simulink model "code_gen_man_bin"  (Simulink 7.5)
settings: Solver=FixedStepDiscrete  SolverMode=SingleTasking  StartTime=0.0  StopTime=10.0  FixedStep=0.01  RelTol=1e-3
InitFcn:
  | boat_constants
values from neighbouring files (symbols this model uses):
  figure8_waypoints = int32([ ... (first row only)    [boat_constants.m]
  InitialPoint = 0    [boat_constants.m]    (also in l2plus.m)
  IPStar = 0    [boat_constants.m]    (also in l2plus.m)
  ISA_g = 9.815    [boat_constants.m]
  MaxDwnPthStar = 1    [boat_constants.m]    (also in l2plus.m)
  OC2max = 49999    [boat_constants.m]    (also in simulation_constants.m)
  sampling_waypoints = int32([ ... (first row only)    [boat_constants.m]
  switchDistance = 4    [boat_constants.m]    (also in l2plus.m)
  T_step = 0.01    [boat_constants.m]    (also in common.m)
  tanIntercept = tan( 45*pi/180 )    [boat_constants.m]    (also in l2plus.m)
  test_waypoints = int32([ ... (first row only)    [boat_constants.m]
  TStar = single(4.5)    [boat_constants.m]    (also in l2plus.m = single(2))
  Turn2Track = 0    [boat_constants.m]    (also in l2plus.m)
  wheelbase = 3.27    [boat_constants.m]
undefined symbols (not defined in the file or in its folder): clearGpsData, clearSensorData, cpInitCommunications, DataEEInitAndClear, DataEEWrite, DiscIntNeverNeededParam, ecan1_buffered_transmit_matlab, ecan1_error_status_matlab, ecan1_init, GetAirData, getGpsData, getRevoData, getSensorData, GetThrottleData, GetWaterData, GetWindData, Init_onlyOnce, Init_Reset, initCalibrationRange, initGps, processNewCommData, processNewGpsData, processNewRevoData, setHilMode, u1, u2, uart1EnqueueStateData, uart2EnqueueActuatorData, y1
libraries: simulink x80, dsPICdrivers x50, uSimLib x4, simulink_need_slupdate x4
(part 6 of 6)

== matlab function Controller/Autonomous Controller/Rudder Command/L2 Plus ref WP1 ==
  data: reset input double; L2Vec output single; waypoints input int16; mode input uint8; Puav input single size=3; Vxyz input single size=3; switchDistance parameter double size=1; ISA_g parameter double; tanIntercept parameter double; MaxDwnPthStar parameter double; Turn2Track parameter double; InitialPoint parameter double; IPStar parameter double; TStar parameter double; as_c output single; i0 output double; i1 output double; WP0 output double; WP1 output double
function [L2Vec, as_c, i0, i1, WP0, WP1] = L2PlusWP1(reset, waypoints, mode, Puav, Vxyz, switchDistance, ...
    ISA_g, tanIntercept, MaxDwnPthStar,Turn2Track,...
    InitialPoint, IPStar, TStar)
%==============================
%     computes bank angle command for following a straight line
%     by creating an aim point that may be more than L2 away 
%     from the UAV. The aim point is (usually) farther along the path 
%     toward WP1 than the UAV, and the intercept
%     angle is less than or equal to a specified value. This limits the intercept
%     angle even when the UAV is within L2 of the path.
%     See L2PlusWP1.m for details
    
%         INPUTS   
%             T1      unit vector WP0-->WP1
%             N1      normal to T1
%             WP0     position of "from" waypoint. only needed to set an InitialPoint
%             WP1     position of WP1, active waypoint
%             Puav    position of UAV
%             Vxyz    Inertial velocity
%             switchDistance distance from WP1 to switch to WP2

%         PARAMETERS
%             ISA_g   gravity
%             tanIntercept  tangent of intercept angle
%             MaxDwnPthStar L2 multiplier to determmine downpath aimpoint
%             Turn2Track    true to turn toward T1 instead of L2
%             InitialPoint  true if no line tracking at first--fly direct to some initial point
%             IPStar        L2 multiplier to determing distance of IP from first WP0
%             Tstar         was called L2Base, time constant of response
%             
%         OUTPUTS
%             phi_c   commanded bank angle (positive is a starboard turn)
%             L2Vec   L2 vector toward aim point
%             as_c    commanded lateral acceleration
%             Groundspeed 
%             IP1     position of IP for plotting purposes. IP1(3) = -999 if no IP exists

    persistent IPActive;  %true if flying toward IP
    persistent IP; % location of initial point

    persistent index_0 index_1; % Store the indices for waypoints 0 & 1 respectively
    persistent direction; % Keep track of the direction for patrol mode
    
    % Make sure we have at least two waypoints
    assert(size(waypoints,1) >= 2);

    % Inititalize to the first waypoint
    if isempty(index_0)
        index_0 = int8(1);
    end
    if isempty(index_1)
        index_1 = int8(2);
    end
    if isempty(direction)
        direction = int8(1);
    end
    
    % Reset the waypoints
    if (reset)
        index_0 = int8(1);
        index_1 = int8(2);
    end
    
    % Select the two current waypoints we're dealing with
    WP0 = single(waypoints(index_0,:)');
    WP1 = single(waypoints(index_1,:)');
    i0 = index_0;
    i1 = index_1;
    
    switchToNextWaypoint = false;
    Pwp1 = single(zeros(3,1));
    Pe_y = single(0);
    Dist2WP1 = single(0);
    MinDownPath = single(0);
    Dist2WPSwitch = single(0);
    L2DownPath = single(0);
    L2ToT = single(zeros(3,1));
    L2Vec = single(zeros(3,1));
    IP1 = single([0; 0;-999]); %signal for no IP
    
    Pne = [Puav(1); Puav(2); 0]; %horizontal position
    Vne = [Vxyz(1); Vxyz(2); 0]; % horizontal velocity
    Groundspeed = norm(Vne);
    L2 = single(TStar*Groundspeed);
    WP0ne = single(zeros(3,1));
    
% Calculate N1 and T1
assert(norm(WP1 - WP0) ~= 0);
T1 = WP1-WP0;
T1 = T1/norm(T1);
N1 = [-T1(2); T1(1); 0];
    
%     initialize IP
    if (isempty(IPActive))
        if (InitialPoint)
%             IP is set relative to the first "from" waypoint
            IPActive = -1;
            IP = [WP0(1); WP0(2); 0] - L2*IPStar*T1;
            
            if (norm(IP-Pne) < .001)
                IPActive = 0;
                IP = single([0; 0; -999]);
            end
        else
            IPActive = 0;
            IP = single([0; 0;-999]); %signal for no IP
        end
    end
    IP1 = IP;
    
    
    if (IPActive)
%         no line tracking, direct to IP
        L2Vec = L2*(IP - Pne)/norm(IP - Pne);
%         check to see if at the IP to terminate this mode
        if norm(IP - Pne) < .1*L2
            IPActive = 0;
        end
    else
         if (Pne(1) < 2)
             IP1 = IP1;
         end
%         IP not active, track WP lines
        WPOne = [WP1(1); WP1(2); 0];
        Pwp1 = Pne - [WP1(1); WP1(2); 0]; % position of UAV relative to WP1
        Pe_y = single(Pwp1'*N1); % cross track error
        Dist2WP1 = -single(Pwp1'*T1); % distance to WP1

%         minimum down path distance for Aim Point intersection on T
%         is determined by the intercept angle but limited 
%         in case of very distant intecepts to MaxDwnPthStar*L2
        MinDownPath = single ( min( abs(Pe_y)/tanIntercept, MaxDwnPthStar*L2)); 
        Dist2WPSwitch = Dist2WP1 - switchDistance;
        if ( abs(Pe_y) > L2 )
    %             Make sure aimpoint is no closer to waypoint than calculated switch point.
            L2DownPath = MinDownPath;
        else
    %             within L2 of T and Dist2WPSwitch >= 0, but limit angle of L2 wrt T
            L2DownPath = (max(MinDownPath, (sqrt( L2^2 - Pe_y^2 ))));
        end
        
        if ( Dist2WPSwitch < 0 )
            switchToNextWaypoint = true;
        end
        
         % vector from Pwp1 to aim point on T1
         L2ToT = single(( Dist2WP1 - L2DownPath )*(-T1) - Pwp1);
         if (norm(L2ToT) < .001)
             L2Vec = L2*T1;
         else
            L2Vec = single(L2*( L2ToT/norm(L2ToT) )); % limit size to L2
         end
    %         L2Vec = L2ToT;
%         dummy statements
    end
    Zprod = single(Vxyz(1)*L2Vec(2) - Vxyz(2)*L2Vec(1)); %Z component of cross product
    sinEta = single(Zprod/(Groundspeed*L2));

    as_c = single(2*Groundspeed^2/(L2)*sinEta);
%         bank angle limits outside of this block
    phi_c = single(atan(as_c/ISA_g));

%         now override bank angle if heading in the wrong direction
    if ( Turn2Track && Dist2WPSwitch > 0 && ~IPActive ) 
%             turn to track not L2, gives min displacement from track
        if ( T1'*Vxyz < 0 )
            if ( Pe_y > 0 )
                phi_c = single(+pi/2);
                as_c = single(99);
            else
                phi_c = single(-pi/2);
                as_c = single(-99);
            end
        end
     else
%           turn toward L2, give min displacement toward WP0
        if ( L2Vec'*Vxyz < 0 )
            if ( sinEta < 0 )
                phi_c = single(-pi/2); 
                as_c = single(-99);
            else
                phi_c = single(+pi/2);
                as_c = single(99);
            end
        end
    end

% Now we process waypoint switching. This relies on the switchTrigger
% value set in the above L2+ controller code.
theEnd = false;
if index_1 + 1 <= size(waypoints,1) && waypoints(index_1+1,1) == -1 ...
                                    && waypoints(index_1+1,2) == -1 ...
                                    && waypoints(index_1+1,3) == -1
    theEnd = true;
end
if switchToNextWaypoint
    switch mode
        case 0 % Halt mode
            if size(waypoints,1) >= index_1 + 1 && ~theEnd
                index_0 = index_1;
                index_1 = index_1 + 1;
            end
        case 1 % Loop mode
            % We either continue moving forward through the waypoints...
            if size(waypoints,1) >= index_1 + 1 && ~theEnd
                index_0 = index_1;
                index_1 = index_1 + 1;
            % Or we wrap-around to the starting waypoint
            else
                index_0 = index_1;
                index_1 = int8(1);
            end
        case 2 % Patrol mode
            if direction == 1 % For the forwards direction
                % We either continue moving forwards through the waypoints...
                if size(waypoints,1) >= index_1 + 1 && ~theEnd
                    index_0 = index_1;
                    index_1 = index_1 + 1;
                % Or we start to go backwards
                else
                    index_0 = index_1;
                    index_1 = index_1 - 1;
                    direction = int8(0);
                end
            elseif direction == 0 % For the reverse direction
                % We either continue moving backwards through the waypoints...
                if index_1 - 1 >= 1
                    index_0 = index_1;
                    index_1 = index_1 - 1;
                % Or we start to go forwards
                else
                    index_0 = index_1;
                    index_1 = index_1 + 1;
                    direction = int8(1);
                end
            end
    end
end

== matlab function Actuator Outputs/To Drive Motor/myMux ==
  data: u1 input double; y output double; u2 input double; u3 input double; u4 input double; u5 input double
function y = myMux(u1, u2, u3, u4, u5)
u5_u16 = uint16(u5);
y = uint16([u1(1); u2(1); u3(1); u4(1); 0; 0; 0; 0;]);

len = length(u5);
if len > 1
    y(5) = bitor(bitshift(u5_u16(1),8),u5_u16(2));
elseif len > 0
    y(5) = u5_u16(1);
end
if len > 3
    y(6) = bitor(bitshift(u5_u16(3),8),u5_u16(4));
elseif len > 2
    y(6) = u5_u16(3);
end
if len > 5
    y(7) = bitor(bitshift(u5_u16(5),8),u5_u16(6));
elseif len > 4
    y(7) = u5_u16(5);
end
if len > 7
    y(8) = bitor(bitshift(u5_u16(7),8),u5_u16(8));
elseif len > 6
    y(8) = u5_u16(7);
end

== matlab function Sensor Inputs/GPS/Unpack sensor data ==
  data: latitude output double; longitude output double; altitude output double; year output double; month output double; day output double; hour output double; minute output double; second output double; cog output double; sog output double; u input uint8; hdop output double; fix output double; satellites output double; newGpsData output double
function [latitude, longitude, altitude, year, month, day, hour, minute, second, cog, sog, hdop, fix, satellites, newGpsData] = unpack(u)
%#eml

latitude = typecast(u(1:4), 'single');
longitude = typecast(u(5:8), 'single');
altitude = typecast(u(9:12), 'single');
year = u(13);
month = u(14);
day = u(15);
hour = u(16);
minute = u(17);
second = u(18);
cog = typecast(u(19:22), 'single');
sog = typecast(u(23:26), 'single');
hdop = typecast(u(27:30), 'single');
fix = u(31);
satellites = u(32);
newGpsData = u(33);

== matlab function Sensor Inputs/Estop detection/Unpack throttle data ==
  data: u input uint8; throttle output double; newData output double
function [throttle, newData] = unpack(u)
%#eml

throttle = typecast(u(1:2), 'int16');
newData = u(3);

== matlab function Sensor Inputs/Toggle ==
  data: u input double; y output double
function y = toggle(u)
%#eml

persistent pre_output;

% Initialize pre_output
if isempty(pre_output)
    pre_output = false;
end

% If we receive the toggle input, toggle
if u
    if pre_output
        pre_output = false;
    else
        pre_output = true;
    end
end

y = pre_output;

== matlab function Controller/Radio Control Inputs1/Detect calibration trigger/Compute Calibration State ==
  data: trigger input boolean; state output uint8; restoredCalibration input double
function state = fcn(trigger, restoredCalibration)
%#eml

persistent countdownTimer transitionCounter internalState;

% Initialize persistent variables
if isempty(countdownTimer)
    countdownTimer = uint8(0);
    transitionCounter = uint8(0);
    
    if restoredCalibration
        internalState = uint8(3);
    else
        internalState = uint8(0);
    end
end

% Do the state processing:
switch internalState
    case 0 % Off
        % When we get a trigger, go into state 1 clearing the timer for use
        if trigger
            transitionCounter = uint8(1);
            internalState = uint8(1);
            countdownTimer = uint8(0);
        end
    case 1 % Transition mode
        % Here we just keep a timer going and once it expires we go back to off,
        % otherwise we count transitions until we've hit 3 then we go to calibration mode.
        countdownTimer = countdownTimer + 1;
        if countdownTimer > 150
            internalState = uint8(0);
        elseif trigger
            transitionCounter = transitionCounter + 1;
        
            % Once we've hit three transitions, we're in calibration mode!
            if transitionCounter == uint8(3)
                internalState = uint8(2);
            end
        end
    case 2 % Calibration mode
        % On the trigger, go into a calibrated mode.
        if trigger
            internalState = uint8(3);
        end
    case 3 % Calibrated
        % When we get a trigger, go into state 4 clearing the timer for use
        if trigger
            transitionCounter = uint8(1);
            internalState = uint8(4);
            countdownTimer = uint8(0);
        end
    case 4 % Transition mode (post-calibration)
        % Here we just keep a timer going and once it expires we go back to calibrated,
        % otherwise we count transitions until we've hit 3 then we go to calibration mode.
        countdownTimer = countdownTimer + 1;
        if countdownTimer > 150
            internalState = uint8(3);
        elseif trigger
            transitionCounter = transitionCounter + 1;
        
            % Once we've hit three transitions, we're in calibration mode!
            if transitionCounter == uint8(3)
                internalState = uint8(2);
            end
        end
end

% Output the internal state
state = internalState;

== matlab function Sensor Inputs/Unpack wind data ==
  data: speed output double; direction output double; newData output double; u input uint8
function [speed, direction, newData] = unpack(u)
%#eml

speed = typecast(u(1:4), 'single');
direction = typecast(u(5:8), 'single');
newData = u(9);

== matlab function Controller/Select current waypoint track ==
  data: reset output double; nextTrack input double; resetTrackNumber input double; test_waypoints parameter double; figure8_waypoints parameter double; sampling_waypoints parameter double; waypoints output double
function [reset, waypoints] = selectTrack(nextTrack, resetTrackNumber, test_waypoints, figure8_waypoints, sampling_waypoints)
%#eml


% Initialize trackNumber.
% This variable is our state, which is the set of waypoints we're navigating
% between.
persistent trackNumber;
if isempty(trackNumber)
    trackNumber = uint8(1);
end

% Here is the logic for switching tracks. trackReset resets the trackNumber
% and nextTrack increments the track number
if resetTrackNumber
    trackNumber = uint8(1);
    reset = true;
elseif nextTrack
    trackNumber = trackNumber + uint8(1);
    if trackNumber > 3
        trackNumber = uint8(1);
    end
    reset = true;
else
    reset = false;
end

% 1 is for the test waypoints, 2 is for the figure eight, and 3 is
% for the data gathering waypoints.
switch trackNumber
    case 1
        waypoints = test_waypoints;
    case 2
        waypoints = figure8_waypoints;
    case 3
        waypoints = sampling_waypoints;
    otherwise
        waypoints = zeros(size(test_waypoints), 'int32');
end

== matlab function Transmit state data via UART1/Pack1 ==
  data: L2 input double; gPos input double; head input double; lPos input double; vel input double; wp0 input double; wp1 input double; y output double; rudder_pot input double; port_limit input double; sb_limit input double; lat input double; lon input double; alt input double; yr input double; mon input double; day input double; hr input double; min input double; sec input double; cog input double; sog input double; hdop input double; fix input double; sat input double; reset input double; load input double; rudder_angle input double; v_rpm input double; status input double; ordering input double; rudderAngleCommand input double; throttleCommand input double; batteryVoltage input double; batteryAmperage input double; lowRudderCalLimit input double; highRudderCalLimit input double; revoHeading input double; revoMagStatus input double; revoPitch input double; revoPitchStatus input double; revoRoll input double; revoRollStatus input double; revoDip input double; revoMagneticMagnitude input double; windSpeed input double; windDirection input double; airTemp input double; airPressure input double; airHumidity input double; waterSpeed input double; waterTemp input double; waterDepth input double
function y = fcn(L2, gPos, head, lPos, vel, wp0, wp1, rudder_pot, port_limit, sb_limit, lat, lon, alt, yr, mon, day, hr, min, sec, cog, sog, hdop, fix, sat, reset, load, rudder_angle, v_rpm, status, ordering, rudderAngleCommand, throttleCommand, batteryVoltage, batteryAmperage, lowRudderCalLimit, highRudderCalLimit, revoHeading, revoMagStatus, revoPitch, revoPitchStatus, revoRoll, revoRollStatus, revoDip, revoMagneticMagnitude, windSpeed, windDirection, airTemp, airPressure, airHumidity, waterSpeed, waterTemp, waterDepth)
%#eml

y = zeros(153, 1, 'uint8');
y(1:4) = packUint32BE(typecast(L2(1),'uint32'));
y(5:8) = packUint32BE(typecast(L2(2),'uint32'));
y(9:12) = packUint32BE(typecast(gPos(1),'uint32'));
y(13:16) = packUint32BE(typecast(gPos(2),'uint32'));
y(17:20) = packUint32BE(typecast(head,'uint32'));
y(21:24) = packUint32BE(typecast(lPos(1),'uint32'));
y(25:28) = packUint32BE(typecast(lPos(2),'uint32'));
y(29:32) = packUint32BE(typecast(vel(1),'uint32'));
y(33:36) = packUint32BE(typecast(vel(2),'uint32'));
y(37:40) = packUint32BE(typecast(wp0(1),'uint32'));
y(41:44) = packUint32BE(typecast(wp0(2),'uint32'));
y(45:48) = packUint32BE(typecast(wp1(1),'uint32'));
y(49:52) = packUint32BE(typecast(wp1(2),'uint32'));
y(53:54) = packUint16BE(rudder_pot);
y(55) = port_limit;
y(56) = sb_limit;
y(57:60) = packUint32BE(typecast(lat,'uint32'));
y(61:64) = packUint32BE(typecast(lon,'uint32'));
y(65:68) = packUint32BE(typecast(alt,'uint32'));
y(69) = yr;
y(70) = mon;
y(71) = day;
y(72) = hr;
y(73) = min;
y(74) = sec;
y(75:78) = packUint32BE(typecast(cog,'uint32'));
y(79:82) = packUint32BE(typecast(sog,'uint32'));
y(83:86) = packUint32BE(typecast(hdop,'uint32'));
y(87) = fix;
y(88) = sat;
y(89) = reset;
y(90) = load;
y(91:94) = packUint32BE(typecast(rudder_angle,'uint32'));
y(95:96) = packUint16BE(typecast(v_rpm,'uint16'));
y(97) = status;
y(98) = ordering;
y(99:102) = packUint32BE(typecast(rudderAngleCommand,'uint32'));
y(103:104) = packUint16BE(typecast(throttleCommand, 'uint16'));
y(105:108) = packUint32BE(typecast(batteryVoltage,'uint32'));
y(109:112) = packUint32BE(typecast(batteryAmperage,'uint32'));
y(113:114) = packUint16BE(typecast(lowRudderCalLimit, 'uint16'));
y(115:116) = packUint16BE(typecast(highRudderCalLimit, 'uint16'));
y(117:120) = packUint32BE(typecast(revoHeading,'uint32'));
y(121) = revoMagStatus;
y(122:125) = packUint32BE(typecast(revoPitch,'uint32'));
y(126) = revoPitchStatus;
y(127:130) = packUint32BE(typecast(revoRoll,'uint32'));
y(131) = revoRollStatus;
y(132:135) = packUint32BE(typecast(revoDip, 'uint32'));
y(136:137) = packUint16BE(typecast(revoMagneticMagnitude,'uint16'));
y(138:139) = packUint16BE(typecast(windSpeed, 'uint16'));
y(140:141) = packUint16BE(typecast(windDirection, 'uint16'));
y(142:143) = packUint16BE(typecast(airTemp, 'uint16'));
y(144:145) = packUint16BE(typecast(airPressure, 'uint16'));
y(146:147) = packUint16BE(typecast(airHumidity, 'uint16'));
y(148:149) = packUint16BE(typecast(waterSpeed, 'uint16'));
y(150:151) = packUint16BE(typecast(waterTemp, 'uint16'));
y(152:153) = packUint16BE(typecast(waterDepth, 'uint16'));

function out = packUint32BE(in)
out = zeros(4, 1, 'uint8');
out(1) = uint8(bitand(bitshift(in,-24),hex2dec('FF')));
out(2) = uint8(bitand(bitshift(in,-16),hex2dec('FF')));
out(3) = uint8(bitand(bitshift(in,-8),hex2dec('FF')));
out(4) = uint8(bitand(in,hex2dec('FF')));

function out = packUint16BE(in)
out = zeros(2, 1, 'uint8');
out(1) = uint8(bitand(bitshift(in,-8),hex2dec('FF')));
out(2) = uint8(bitand(in,hex2dec('FF')));

== matlab function Controller/Radio Control Inputs1/If Action Subsystem1/Map into range ==
  data: mappedValue output int32; val input int32; in_min input int32; in_max input int32; out_min input int32; out_max input int32
function mappedValue = map(val, in_min, in_max, out_min, out_max)
%#eml
% Pulled from: http://www.arduino.cc/cgi-bin/yabb2/YaBB.pl?num=1289758376, first post
% This is a basic integer implementation of a map() function.
% NOTE: There can be integer overflow in the first multiplication.

  mappedValue = (val - in_min) * (out_max - out_min) / (in_max - in_min) + out_min;

end

== matlab function Controller/Radio Control Inputs1/If Action Subsystem3/Map into range ==
  data: mappedValue output int32; val input int32; in_min input int32; in_max input int32; out_min input int32; out_max input int32
function mappedValue = map(val, in_min, in_max, out_min, out_max)
%#eml
% Pulled from: http://www.arduino.cc/cgi-bin/yabb2/YaBB.pl?num=1289758376, first post
% This is a basic integer implementation of a map() function.
% NOTE: There can be integer overflow in the first multiplication.

  mappedValue = (val - in_min) * (out_max - out_min) / (in_max - in_min) + out_min;

end

== matlab function Transmit state data via UART1/Embedded MATLAB Function ==
  data: T input double; wp0 output double; i0 input double; i1 input double; wp1 output double
function [wp0, wp1] = fcn(T, i0, i1)
%#eml

wp0 = T(i0,:);
wp1 = T(i1,:);

== matlab function Controller/Radio Control Inputs1/If Action Subsystem5/Map into range ==
  data: mappedValue output int32; val input int32; in_min input int32; in_max input int32; out_min input int32; out_max input int32
function mappedValue = map(val, in_min, in_max, out_min, out_max)
%#eml
% Pulled from: http://www.arduino.cc/cgi-bin/yabb2/YaBB.pl?num=1289758376, first post
% This is a basic integer implementation of a map() function.
% NOTE: There can be integer overflow in the first multiplication.

  mappedValue = (val - in_min) * (out_max - out_min) / (in_max - in_min) + out_min;

end

== matlab function Controller/Autonomous Controller/Throttle Command/Mux Everything/Select data packet ==
  data: y output double; dis input double; en input double
function y = fcn(dis, en)
% This block controls the switch selecting between enable, 
% disable, and speed commands. If disable and enable are
% both set high, disable overrides anything else.

y = uint8(3);
if dis == 1
    y = uint8(1);
elseif en == 1
    y = uint8(2);
end

== matlab function Transmit state data via UART1/Build HIL sentence/Pack ==
  data: a input double; y output double; b input double; c input double; d input double; e input double; f input double
function y = fcn(a, b, c, d, e, f)
%#eml

y = zeros(length(a)+length(b)+length(c)+length(d)+length(e)+length(f), 1, 'uint8');
y(1) = a;
y(2) = b;
y(3:157) = c;
y(158) = d;
y(159) = e;
y(160) = f;

== matlab function Controller/Radio Control Inputs1/autoMode State Checker ==
  data: rcInput input double; y output double; HIL input double
function y  = fcn(rcInput, HIL)
%#eml

% Initialize a persistent state variable that initializes to -1, the startup
% state value.
persistent internalState;
if isempty(internalState)
    internalState = int8(-1);
end

% Implement the state machine.
switch internalState
    case -1 % Startup
        if rcInput ~= 0
            if rcInput > 7000
                internalState = int8(0);
            else
                internalState = int8(1);
            end
        elseif HIL
            internalState = int8(1);
        end
    case 0 % Manual mode
        if rcInput ~= 0
            if rcInput > 7000
                internalState = int8(0);
            else
                internalState = int8(1);
            end
        elseif HIL
            internalState = int8(1);
        end
    case 1 % Autonomous mode
        if rcInput ~= 0
            if rcInput > 7000
                internalState = int8(0);
            else
                internalState = int8(1);
            end
        end
end
    
% Here the current autonomous state is output as either 1:"on" or 0:"off"
if internalState == int8(1)
    y = true;
else
    y = false;
end

== matlab function Sensor Inputs/Toggle1 ==
  data: u input double; y output double
function y = toggle(u)
%#eml

persistent pre_output;

% Initialize pre_output
if isempty(pre_output)
    pre_output = false;
end

% If we receive the toggle input, toggle
if u
    if pre_output
        pre_output = false;
    else
        pre_output = true;
    end
end

y = pre_output;

== matlab function Sensor Inputs/Unpack air data ==
  data: temp output double; pressure output double; humidity output double; newData output double; u input uint8
function [temp, pressure, humidity, newData] = unpack(u)
%#eml

temp = typecast(u(1:4), 'single');
pressure = typecast(u(5:8), 'single');
humidity = typecast(u(9:12), 'single');
newData = u(13);

== matlab function Controller/Rudder sensor calibration/Run rudder for calibration ==
  data: rudderAngle output double; trigger input double; reset input double; rudderPot input double; rudderPortLimit input double; rudderSbLimit input double; step output double; dir output double; throttle output double; mode output double; lowLimit output double; highLimit output double
function [rudderAngle, step, dir, throttle, mode, lowLimit, highLimit] = calibrate(trigger, reset, rudderPot, rudderPortLimit, rudderSbLimit)
    %#eml

    % cal_state stores which state we're in. 0 indicates no calibration, 2 means
    % calibrating the port limit, 1 means calibration the starboard limit
    persistent cal_state direction run drive calibrating low_side high_side lastInput offset calibrated;
    if isempty(cal_state) || reset
        cal_state = uint8(0);      % State machine state
        direction = false;         % Commanded rudder direction (true for port, false for starboard)
        run = false;               % Commanded rudder enable
        calibrating = false;       % Calibrating when true
        drive = true;              % Drive is initialized to true here such that it will trigger a transition at the start and end of the calibration control code.
        low_side = int32(-1);      % The lowest limit read from the potentiometer
        high_side = int32(-1);     % The highest limit read from the potentiometer
        lastInput = int32(-10000); % The last rudder potentiometer value
        offset = int32(0);         % Used to correct rudder position wrap-around
        calibrated = false;        % Whether the rudder is calibrated
    end

    if trigger
        calibrating = ~calibrating;
    end
    
    % Here we track transitions. On a high->low transition start adding 1023
    % and on a low->high transition don't add anything. It "centers" the input
    % range around 1023.
    input = int32(rudderPot);
    if lastInput == uint32(-10000)
        lastInput = input;
    end
    jump = input - lastInput;
    if jump > 1000
        offset = int32(0);
    elseif jump < -1000
        offset = int32(1023);
    end

    % We record the last input BEFORE it's offset. This fixes situations where
    % we're comparing data before and after the very first transition.
    lastInput = input;

    % Apply any offset that should be there.
    input = input + offset;

    % We perform the output generation here, before the state machine, as the rudderAngle is required for the last state.
    highLimit = int16(high_side);
    lowLimit = int16(low_side);
    if calibrated
        rudderAngle = pot_to_rads(rudderPot, high_side, low_side);
    else
        % Return 0 when we can't actually determine the rudder position
        rudderAngle = single(0);
    end

    if cal_state == 0 % Waiting for calibration trigger
        if trigger
            cal_state = uint8(6);
            low_side = int32(-1);
            high_side = int32(-1);
            calibrated = false;
            drive = false;
        end
    elseif cal_state == 6 % Initial calibration mode
        if ~calibrating % Reset if calibration is disabled
            cal_state = uint8(0);
            run = false;
            drive = true;
        elseif rudderSbLimit % If the starboard limit is active, go to port first
            cal_state = uint8(5);
            run = true;
            direction = true;
        else % Default to heading towards the center
            run = true;
            if rudderPot > 450
                % Head to port if on the starboard side
                direction = true;
                cal_state = uint8(5);
            else
                % Head to starboard if on the port side
                direction = false;
                cal_state = uint8(4);
            end
        end
    elseif cal_state == 5 % Calibrating the first limit (port)
        if ~calibrating % Reset if calibration is disabled
            cal_state = uint8(0);
            run = false;
            drive = true;
        elseif rudderPortLimit % If we've hit the limit, we're done here
            low_side = input;

            % If the high_side limit is less than the low_side one, we add 1023
            % assuming that it's a valid value (ie. ~= -1).
            if high_side < low_side && high_side ~= -1
                high_side = high_side + 1023;
            end
            
            cal_state = uint8(2);
            direction = false;
        end
    elseif cal_state == 4 % Calibrating the first limit (starboard)
        if ~calibrating % Reset if calibration is disabled
            cal_state = uint8(0);
            run = false;
            drive = true;
        elseif rudderSbLimit % If we've hit the limit, we're done here
            high_side = input;

            % If the high_side limit is less than the low_side one, we add 1023
            % assuming that it's a valid value (ie. ~= -1).
            if high_side < low_side && high_side ~= -1
                high_side = high_side + 1023;
            end
        
            cal_state = uint8(3);
            direction = true;
        end
    elseif cal_state == 3 % Last limit calibration (port)
        if ~calibrating % Reset if calibration is disabled
            cal_state = uint8(0);
            run = false;
            drive = true;
        elseif rudderPortLimit % If we've hit the port limit then we're done calibrating, so we recenter the rudder.
            low_side = input;

            % If the high_side limit is less than the low_side one, we add 1023
            % assuming that it's a valid value (ie. ~= -1).
            if high_side < low_side && high_side ~= -1
                high_side = high_side + 1023;
            end
            
            calibrated = true;
            cal_state = uint8(1);
            direction = false;
        end
    elseif cal_state == 2 % Last limit calibration (starboard)
        if ~calibrating % Reset if calibration is disabled
            cal_state = uint8(0);
            run = false;
            drive = true;
        elseif rudderSbLimit % If we've hit the starboard limit then we're done calibrating, so we recenter the rudder.
            high_side = input;

            % If the high_side limit is less than the low_side one, we add 1023
            % assuming that it's a valid value (ie. ~= -1).
            if high_side < low_side && high_side ~= -1
                high_side = high_side + 1023;
            end
            
            calibrated = true;
            cal_state = uint8(1);
            direction = true;
        end
    elseif cal_state == 1 % Center the rudder
        if ~calibrating % Reset if calibration is disabled
            cal_state = uint8(0);
            run = false;
            drive = true;
        elseif abs(rudderAngle) < 0.1 % If we're close to the center, stop commanding the rudder. Set to 0.1 to account for delay
            cal_state = uint8(0);
            run = false;
            drive = true;
            calibrating = false;
        end
    end
    
    % Specify the calibration mode using a bitmask:
    % Bit 0: Calibrating
    % Bit 1: Calibrated
    mode = bitor(uint8(calibrating), bitshift(uint8(calibrated), 1));
    
    % Set the rest of the outputs
    step = run;
    dir = direction;
    throttle = drive;
end

function [rads] = pot_to_rads(input, high_side, low_side)
    %#eml
    % This function converts the potentiometer reading from the boat's rudder sensors
    % to a value in degrees. It relies on each limit being hit to set the bounds on
    % the rudder sensor value and then maps that value from that range into the new
    % range of -.07854 to .07854 (+-45 deg). It is loosely based off of the integer
    % mapping function at: http://www.arduino.cc/cgi-bin/yabb2/YaBB.pl?num=1289758376

    % Prepare our input. Here we subtract the baseline 'low_side' value off of
    % the input so we start with a range from [0..high_side-lowside] and map it
    % into the output range of 45 degrees.
    in_max = high_side - low_side;
    val = int32(input) - low_side;

    % Do the actual conversion reversing the range and mapping it into [.7854:-0.7854]
    rads = (0.5 - single(val)/single(in_max))*2*0.7854;

    % Finally cap the value to +- our range to prevent odd errors later.
    if rads > 0.7854
        rads = single(0.7854);
    elseif rads < -0.7854
        rads = single(-0.7854);
    end
end

== matlab function Sensor Inputs/Unpack water data ==
  data: speed output double; temp output double; depth output double; newData output double; u input uint8
function [speed, temp, depth, newData] = unpack(u)
%#eml

speed = typecast(u(1:4), 'single');
temp = typecast(u(5:8), 'single');
depth = typecast(u(9:12), 'single');
newData = u(13);

== matlab function Controller/Radio Control Inputs1/Clear to 0 if Disconnect/Set the throttle to 0 if it's only a heartbeat ==
  data: u input double; y output double
function y = fcn(u)
%#eml

if u < int16(4700)
    y = int16(0);
else
    y = u;
end

== matlab function Controller/Radio Control Inputs1/If Action Subsystem1/Add binning ==
  data: manualRudderAngle input double; newManualRudderAngle output double
function newManualRudderAngle  = fcn(manualRudderAngle)
%#eml
    % This function converts the continuous input of the rudder angle
    % command into a up/down/no change control. This allows for the commanded
    % rudder value to remain constant, which is useful for doing rudder
    % tests.
    
    % Once the input is above 25 or below -25 degrees (in radians) then a
    % counter starts for 25 timesteps (so .25s total) to see if the rudder
    % angle should change. Then it waits until the commanded angle resets
    % to around 0 (between +- 10 degrees) and then another transition can
    % occur.
    
    % This function relies on a 4-state FSM. It follows the general pattern
    % of 0-1-3 or 0-2-3 on success. 0 is the initial state, 1 and 2 are the
    % same, just moving in different directions, and 3 is the cleanup.

    % Keep a counter going of how long they have requested a bin transition
    persistent transitionCounter state nullTransitionCounter;
    if isempty(transitionCounter)
        transitionCounter = uint8(0);
        nullTransitionCounter = uint8(0);
        state = uint8(0);
    end

    % Store the mapped rudder angles for each bin
    binAngles = single([-45 -33 -22 -11 0 11 22 33 45]*pi/180);

    % Keep track of which bin we're in so that hysteresis can be done. This is
    % NOT a stateless algorithm. We initialize into the 0th bin (which is 1 in
    % this case because of Matlab's 1 indexing).
    persistent bin;
    if isempty(bin)
        bin = uint8(5);
    end

    switch state
        case 0
            if manualRudderAngle > 25*pi/180;
                transitionCounter = uint8(0);
                state = uint8(1);
            elseif manualRudderAngle < -25*pi/180;
                transitionCounter = uint8(0);
                state = uint8(2);
            end
        case 1
            % If the user is still indicating a transition, keep counting.
            % Otherwise record null transition commands.
            if manualRudderAngle > 25*pi/180;
                transitionCounter = transitionCounter + uint8(1);
            else
                nullTransitionCounter = nullTransitionCounter + uint8(1);
            end
            
            % Either transition if possible and requested or fail out after
            % having encountered too many timesteps without a request.
            if transitionCounter > 25
                if bin + uint8(1) <= length(binAngles)
                    bin = bin + uint8(1);
                end
                state = uint8(3);
            elseif nullTransitionCounter > 8
                state = uint8(3);
            end
        case 2
            if manualRudderAngle < -25*pi/180;
                transitionCounter = transitionCounter + uint8(1);
            else
                nullTransitionCounter = nullTransitionCounter + uint8(1);
            end
            if transitionCounter > 25
                if bin - uint8(1) > 0
                    bin = bin - uint8(1);
                end
                state = uint8(3);
            elseif nullTransitionCounter > 8
                state = uint8(3);
            end
        case 3
            if manualRudderAngle < 10*pi/180 && manualRudderAngle > -10*pi/180
                state = uint8(0);
                nullTransitionCounter = uint8(0);
            end
    end
    
    newManualRudderAngle = binAngles(bin);
end
